simulink model "sim1"  (R2022b)
settings: Solver=VariableStepAuto  StartTime=0.0  StopTime=10  RelTol=1e-3
settings Model: Creator=acer  LastModifiedBy=acer

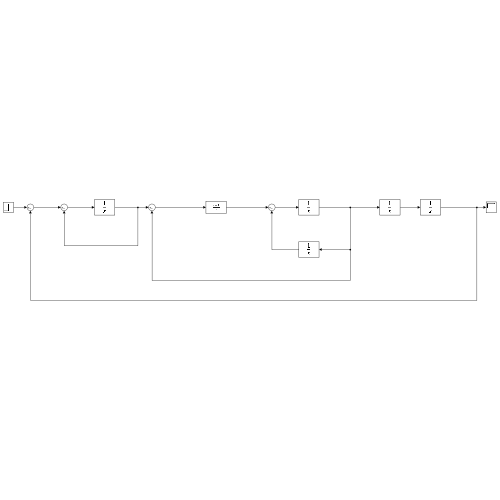
[thumbnail: Simulink's stored preview of the top-level diagram]
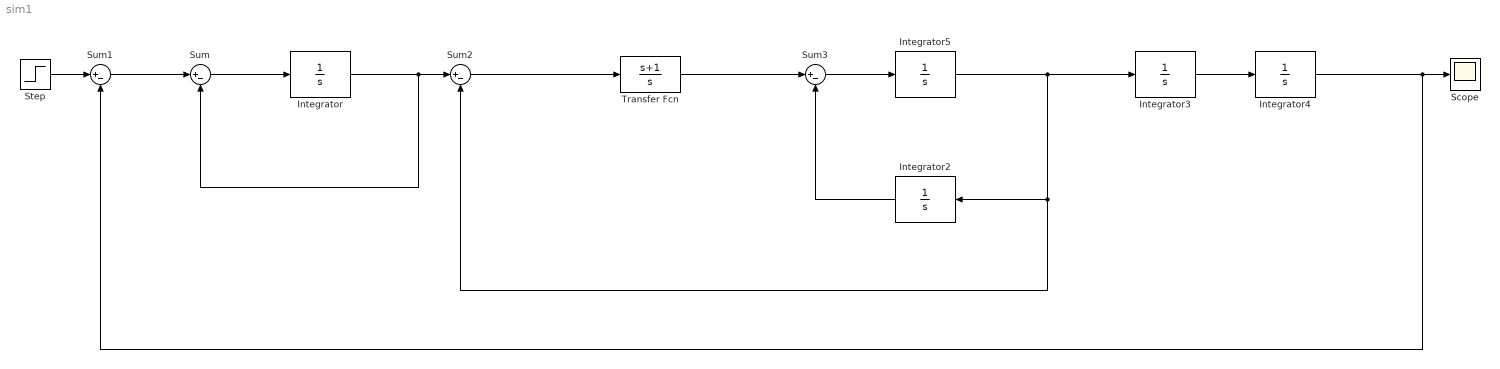
== system sim1 ==
  Integrator{,2..5} (5 alike) : Integrator
  Scope : Scope
  Step : Step  SampleTime=0
  Sum{,1..3} (4 alike) : Sum  Inputs=|+-
  Transfer Fcn : TransferFcn  Numerator=[1,1]  Denominator=[1 0]
  wires:
  Sum/1 -> Integrator/1
  Step/1 -> Sum1/1
  Integrator/1 -> Sum/2, Sum2/1
  Sum3/1 -> Integrator5/1
  Integrator3/1 -> Integrator4/1
  Sum1/1 -> Sum/1
  Integrator2/1 -> Sum3/2
  Sum2/1 -> Transfer Fcn/1
  Transfer Fcn/1 -> Sum3/1
  Integrator5/1 -> Integrator3/1, Sum2/2, Integrator2/1
  Integrator4/1 -> Sum1/2, Scope/1
